simulink model "Trial_BOARD"  (R2015a)
settings: Solver=ode3  StartTime=0.0  StopTime=inf  FixedStep=0.001  RelTol=1e-3
libraries: PoliArd x23, simulink x2
settings Model: ExtModeTrigDuration=2  Creator=User  LastModifiedBy=user
settings OptimizationCC: OptimizeModelRefInitCode=on  LifeSpan=1
settings DebuggingCC: UnderspecifiedInitializationDetection=Classic  MergeDetectMultiDrivingBlocksExec=none
settings HardwareCC: ProdLargestAtomicInteger=Long  ProdLargestAtomicFloat=Double  ProdEndianess=LittleEndian  ProdHWDeviceType=ARM Compatible->ARM Cortex
settings RTWCC: SystemTargetFile=realtime.tlc  GenerateMakefile=off  TemplateMakefile=realtime.tmf  Description=Run on Target Hardware  RTWVerbose=off
settings ERTTargetCC: CombineOutputUpdateFcns=off  ExtModeTransport=3  ExtModeMexFile=ext_serial_win32_comm_rtt  ExtModeMexArgs=0 1 9600  InlinedParameterPlacement=Hierarchical  ERTSrcFileBannerTemplate=realtime_code_template.cgt  ERTHdrFileBannerTemplate=realtime_code_template.cgt  ERTDataSrcFileTemplate=realtime_code_template.cgt  ERTDataHdrFileTemplate=realtime_code_template.cgt  ERTCustomFileTemplate=realtime_file_process.tlc

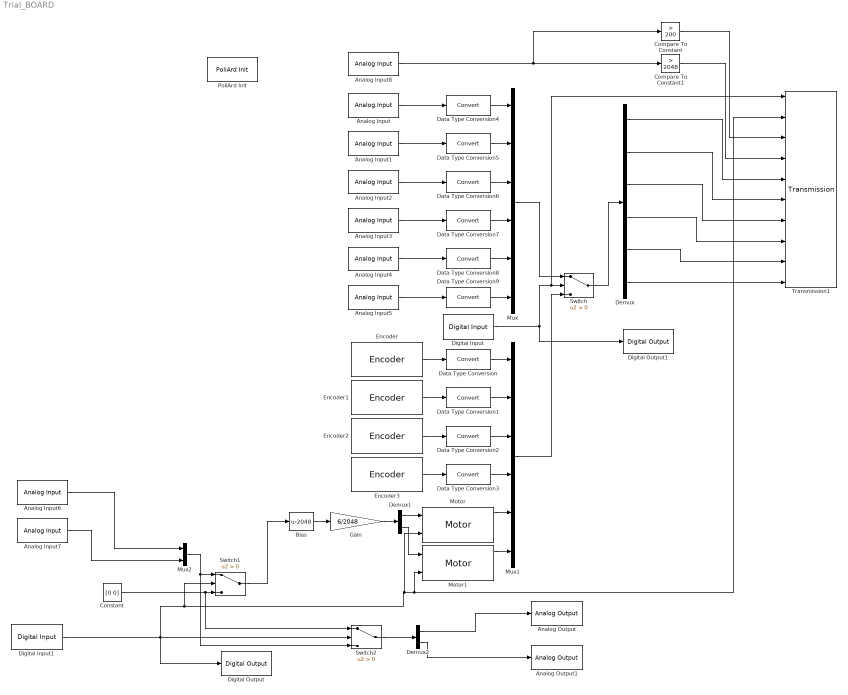
== system Trial_BOARD ==
  Analog Input : PoliArd/Analog Input  AIpin_mask=1  AIsample=-1
  Analog Input1 : PoliArd/Analog Input  AIpin_mask=2  AIsample=-1
  Analog Input2 : PoliArd/Analog Input  AIpin_mask=3  AIsample=-1
  Analog Input3 : PoliArd/Analog Input  AIpin_mask=4  AIsample=-1
  Analog Input4 : PoliArd/Analog Input  AIpin_mask=5  AIsample=-1
  Analog Input5 : PoliArd/Analog Input  AIpin_mask=6  AIsample=-1
  Analog Input6 : PoliArd/Analog Input  AIpin_mask=8  AIsample=-1
  Analog Input7 : PoliArd/Analog Input  AIpin_mask=9  AIsample=-1
  Analog Input8 : PoliArd/Analog Input  AIpin_mask=7  AIsample=-1
  Analog Output : PoliArd/Analog Output  DAC_pin_mask=1
  Analog Output1 : PoliArd/Analog Output  DAC_pin_mask=2
  Bias : Bias  Bias=-2048
  Compare To Constant : simulink/Logic and Bit Operations/Compare To Constant  relop=>  const=200  OutDataTypeStr=boolean
  Compare To Constant1 : simulink/Logic and Bit Operations/Compare To Constant  relop=>  const=2048  OutDataTypeStr=boolean
  Constant : Constant  Value=[0 0]
  Data Type Conversion{,1..9} (10 alike) : DataTypeConversion
  Demux : Demux  Outputs=6
  Demux1 : Demux  Outputs=2
  Demux2 : Demux  Outputs=2
  Digital Input : PoliArd/Digital Input  DI_pin=2  DIsample=-1
  Digital Input1 : PoliArd/Digital Input  DI_pin=3  DIsample=-1
  Digital Output : PoliArd/Digital Output  DO_pin=2
  Digital Output1 : PoliArd/Digital Output  DO_pin=1
  Encoder : PoliArd/Encoder  EncoderID=1  dt_enc=-1
  Encoder1 : PoliArd/Encoder  EncoderID=2  dt_enc=-1
  Encoder2 : PoliArd/Encoder  EncoderID=3  dt_enc=-1
  Encoder3 : PoliArd/Encoder  EncoderID=4  dt_enc=-1
  Gain : Gain  Gain=6/2048
  Motor : PoliArd/Motor  MotorID=1  DC_bus_mask=12  dt_mot=-1
  Motor1 : PoliArd/Motor  MotorID=2  DC_bus_mask=12  dt_mot=-1
  Mux : Mux  Inputs=6
  Mux1 : Mux  Inputs=6
  Mux2 : Mux  Inputs=2
  PoliArd Init : PoliArd/PoliArd Init
  Switch : Switch  Criteria=u2 > Threshold
  Switch1 : Switch  Criteria=u2 > Threshold
  Switch2 : Switch  Criteria=u2 > Threshold
  Transmission1 : PoliArd/Transmission  sample_freq=100  sig_to_send=6
  wires:
  Demux/2 -> Transmission1/6
  Demux/3 -> Transmission1/7
  Demux/1 -> Transmission1/5
  Demux/4 -> Transmission1/8
  Demux/5 -> Transmission1/9
  Demux/6 -> Transmission1/10
  Mux/1 -> Switch/1
  Switch/1 -> Demux/1
  Digital Input/1 -> Digital Output1/1, Transmission1/1, Switch/2
  Mux1/1 -> Switch/3
  Encoder/1 -> Data Type Conversion/1
  Encoder1/1 -> Data Type Conversion1/1
  Encoder2/1 -> Data Type Conversion2/1
  Encoder3/1 -> Data Type Conversion3/1
  Motor/1 -> Mux1/5
  Motor1/1 -> Mux1/6
  Analog Input6/1 -> Mux2/1
  Analog Input7/1 -> Mux2/2
  Mux2/1 -> Switch2/3, Switch1/1
  Digital Input1/1 -> Switch2/2, Digital Output/1, Transmission1/2, Motor1/2, Motor/2, Switch1/2
  Demux1/1 -> Motor/1
  Demux1/2 -> Motor1/1
  Constant/1 -> Switch2/1, Switch1/3
  Analog Input5/1 -> Data Type Conversion9/1
  Analog Input4/1 -> Data Type Conversion8/1
  Analog Input3/1 -> Data Type Conversion7/1
  Analog Input2/1 -> Data Type Conversion6/1
  Analog Input1/1 -> Data Type Conversion5/1
  Analog Input/1 -> Data Type Conversion4/1
  Data Type Conversion/1 -> Mux1/1
  Data Type Conversion1/1 -> Mux1/2
  Data Type Conversion2/1 -> Mux1/3
  Data Type Conversion3/1 -> Mux1/4
  Data Type Conversion4/1 -> Mux/1
  Data Type Conversion5/1 -> Mux/2
  Data Type Conversion6/1 -> Mux/3
  Data Type Conversion7/1 -> Mux/4
  Data Type Conversion8/1 -> Mux/5
  Data Type Conversion9/1 -> Mux/6
  Switch2/1 -> Demux2/1
  Compare To Constant1/1 -> Transmission1/4
  Compare To Constant/1 -> Transmission1/3
  Analog Input8/1 -> Compare To Constant1/1, Compare To Constant/1
  Bias/1 -> Gain/1
  Gain/1 -> Demux1/1
  Switch1/1 -> Bias/1
  Demux2/2 -> Analog Output1/1
  Demux2/1 -> Analog Output/1
